simulink model "sm_boom_lift_crawler_test_jib_hydr_1D"  (R2026a)
settings: Solver=ode23t  StopTime=tVec.StopTime  MaxStep=2  AbsTol=1e-4
PostLoadFcn:
  | sm_boom_lift_crawler_settest('jib test')
StartFcn:
  | tic;
StopFcn:
  | Elapsed_Sim_Time = toc;
  | %disp(['Elapsed Sim Time = ' num2str(Elapsed_Sim_Time)]);
undefined symbols (not defined in the file): oVec, tVec
libraries: fl_lib x9, nesl_utility x6, sdl_lib x1, sm_boom_lift_crawler_lib_actuators x1, sm_boom_lift_crawler_lib x1
Description:
  | Copyright 2025-2026 The MathWorks, Inc.
settings Model: Creator=smiller  LastModifiedBy=smiller
settings SolverCC: MaxConsecutiveMinStep=5
settings DataIOCC: SignalLoggingName=logsout_sm_boom_lift_crawler
settings SimscapeCC: SimscapeNominalValues="[{\"value\":\"1\",\"unit\":\"A\"},{\"value\":\"nomval_psi\",\"unit\":\"psi\"},{\"value\":\"1\",\"unit\":\"cm^2\"},{\"value\":\"nomval_cmv3_s\",\"unit\":\"cm^3/s\"},{\"value\":\"1\",\"unit\":\"kJ/kg\"},{\"value\":\"1\",\"unit\":\"kW\"},{\"value\":\"1\",\"unit\":\"l\"},{\"value\":\"nomval_N\",\"unit\":\"N\"},{\"value\":\"nomval_Nm\",\"unit\":\"N*m\"},{\"value\":\"1\",\"unit\":\"V\"}]"  SimscapeLogName=simlog_sm_boom_lift_crawler  SimscapeLogLimitData=off  SimscapeLogDataHistory=5000.0  SimscapeUseOperatingPoints=on  SimscapeOperatingPoint=op_jib_hydr_1D

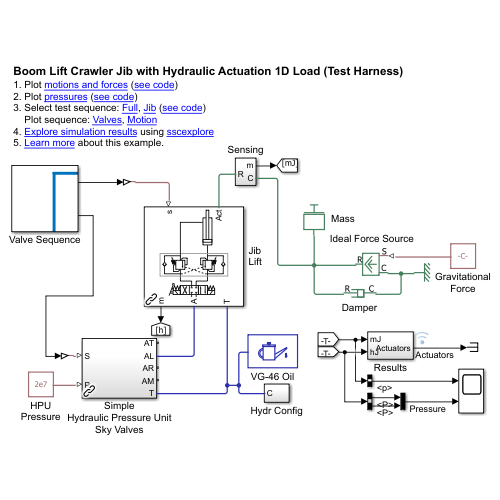
[thumbnail: Simulink's stored preview of the top-level diagram]
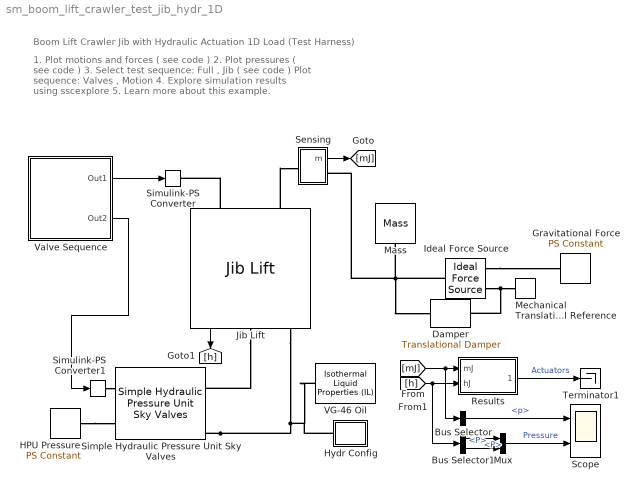
== system sm_boom_lift_crawler_test_jib_hydr_1D ==
  note: Boom Lift Crawler Jib with Hydraulic Actuation 1D Load (Test Harness)
  note: 1. Plot motions and forces ( see code )
      | 2. Plot pressures ( see code )
      | 3. Select test sequence: Full , Jib ( see code )
      | Plot sequence: Valves , Motion
      | 4. Explore simulation results using sscexplore
      | 5. Learn more about this example.
  Bus Selector : BusSelector  OutputSignals=p
  Bus Selector1 : BusSelector  OutputSignals=A.P,B.P
  Damper : sdl_lib/Couplings & Drives/Springs & Dampers/Translational Damper  D=100 N/(m/s)  thermal_port=simscape.enum.thermaleffects.omit  thermal_mass=50 kJ/K  temperature_specify=off  temperature_priority=High  temperature=300 K  temperature_nominal_specify=off  temperature_nominal_value=1  temperature_nominal_unit=K
  Gravitational Force : fl_lib/Physical Signals/Sources/PS Constant  constant=9.8*163
  HPU Pressure : fl_lib/Physical Signals/Sources/PS Constant  constant=2e7 Pa
  Hydr Config : Subsystem
  Ideal Force Source : fl_lib/Mechanical/Mechanical Sources/Ideal Force Source
  Jib Lift : sm_boom_lift_crawler_lib_actuators/Actuators/Sky Manifold/Sky Valves II/Jib Lift  SystemSampleTime=-1  VariantActivationTime=update diagram  EmptyChoice=off  PassThrough=off  PassThroughVariantControl=(default)  EmptyChoiceVariantControl=(default)  AllowFlexibleInterface=on  Latency=0  AutoFrameSizeCalculation=off
  Mass : fl_lib/Mechanical/Translational Elements/Mass  mass=163 kg  num_ports=foundation.enum.numPorts2.one  v_specify=off  v_priority=High  v=0 m/s  v_nominal_specify=off  v_nominal_value=1  v_nominal_unit=m/s  f_specify=off  f_priority=None  f=0 N  f_nominal_specify=off  f_nominal_value=1  f_nominal_unit=N
  Mechanical Translational Reference : fl_lib/Mechanical/Translational Elements/Mechanical Translational Reference
  Mux : Mux  Inputs=2
  Results : Subsystem
  Scope : Scope  NumInputPorts=2
      settings: ActiveDisplayYMinimum=-0.05926  ActiveDisplayYMaximum=0.46698
  Sensing : Subsystem
  Simple Hydraulic Pressure Unit Sky Valves : sm_boom_lift_crawler_lib/Simple Hydraulic Pressure Unit Sky Valves  SystemSampleTime=-1  VariantActivationTime=update diagram  EmptyChoice=off  PassThrough=off  PassThroughVariantControl=(default)  EmptyChoiceVariantControl=(default)  AllowFlexibleInterface=on  Latency=0  AutoFrameSizeCalculation=off
  Simulink-PS Converter : nesl_utility/Simulink-PS Converter  PhysicalDomain=network_engine_domain  SubClassName=ps_input  LeftPortType=input  RightPortType=output  PseudoPeriodic=off  Frequencies=[]  NoiseDistribution=none  NoiseParameters=[]  Unit=1  AffineConversion=off  FilteringAndDerivatives=provide  SimscapeFilterOrder=1  InputFilterTimeConstant=0.001  UdotUserProvided=0
  Simulink-PS Converter1 : nesl_utility/Simulink-PS Converter  PhysicalDomain=network_engine_domain  SubClassName=ps_input  LeftPortType=input  RightPortType=output  PseudoPeriodic=off  Frequencies=[]  NoiseDistribution=none  NoiseParameters=[]  Unit=1  AffineConversion=off  FilteringAndDerivatives=provide  SimscapeFilterOrder=1  InputFilterTimeConstant=0.001  UdotUserProvided=0
  Terminator1 : Terminator
  VG-46 Oil : fl_lib/Isothermal Liquid/Utilities/Isothermal Liquid Properties (IL)  rho_L_atm=867.346 kg/m^3  bulk_modulus_model=foundation.enum.bulk_modulus_model.const  beta_gain=6  beta_L_atm=1.48150e+09 Pa  nu_atm=(45.7333)*(1) cSt  p_atm=0.101325 MPa  p_min=1 Pa  properties_range_check=simscape.enum.assert.action.error  air_fraction=ratio_dissolved_air  polytropic_index=1.0  rho_g_atm=1.225 kg/m^3  air_dissolution_model=simscape.enum.onoff.off  p_crit=3 MPa
  Valve Sequence : Subsystem
      mask Display: image('sm_boom_lift_crawler_valve_seq_outputonly.svg');
  wires:
  [h] -> Bus Selector1/1, Results/2(hJ)
  Valve Sequence/2(Out2) -> Simulink-PS Converter1/1
  Valve Sequence/1(Out1) -> Simulink-PS Converter/1
  Mux/1 -> Scope/2  "Pressure"
  Bus Selector1/2 -> Mux/2  "<P>"
  Sensing/1(m) -> [mJ]
  Bus Selector1/1 -> Mux/1  "<P>"
  [mJ] -> Bus Selector/1, Results/1(mJ)
  Results/1(Actuators) -> Terminator1/1  "Actuators"
  Jib Lift/1 -> [h]
  Bus Selector/1 -> Scope/1  "<p>"
  connections:
  Ideal Force Source/LConn1 -- Mass/LConn1 -- Sensing/RConn1 -- Damper/LConn1
  Mechanical Translational Reference/LConn1 -- Ideal Force Source/RConn2 -- Damper/RConn1
  Simple Hydraulic Pressure Unit Sky Valves/RConn5 -- Jib Lift/RConn2 -- VG-46 Oil/RConn1 -- Hydr Config/RConn1
  Ideal Force Source/RConn1 -- Gravitational Force/RConn1
  HPU Pressure/RConn1 -- Simple Hydraulic Pressure Unit Sky Valves/LConn2
  Simulink-PS Converter1/RConn1 -- Simple Hydraulic Pressure Unit Sky Valves/LConn1
  Jib Lift/RConn1 -- Simple Hydraulic Pressure Unit Sky Valves/RConn2
  Jib Lift/LConn2 -- Sensing/LConn1
  Jib Lift/LConn1 -- Simulink-PS Converter/RConn1

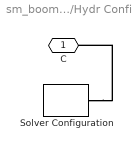
== system sm_boom_lift_crawler_test_jib_hydr_1D/Hydr Config ==
  Solver Configuration : nesl_utility/Solver Configuration  PhysicalDomain=network_engine_domain  SubClassName=solver  LeftPortType=input  RightPortType=generic  Tones=[]  Harmonics=[]  SimulateNoise=off  Profile=off  UseLocalSampling=off  EnableSwitchedLinearOptims=on  FrequencyDomain=off  UseCCode=off  RelTol=0.001  AbsTol=1e-06  MinStep=1e-09  ToWorkspace=off  RevertToSquareIcSolve=off  NumHomotopyIterations=100  PhasorMode=off  PhasorModeNumHarmonics=1  ConsistencySolver=NEWTON_FTOL  CanonicalOrdering=UNORDERED  OptimizeIntermediates=UNOPTIMIZED  IndexReductionMethod=DerivativeReplacement  DoDC=off  ResidualTolerance=1e-9  ConsistencyTolSource=GLOBAL  ConsistencyAbsTol=0.001  ConsistencyRelTol=0.001  ConsistencyTolFactor=0.001  UseLocalSolver=off  LocalSolverChoice=NE_BACKWARD_EULER_ADVANCER  ResolveIndetEquations=on  FunctionEvalNumThread=1  LocalSolverSampleTime=2e-3  DoFixedCost=off  MaxNonlinIter=5  MaxModeIter=2  ComputeImpulses=off  ImpulseIterations=2  LinearAlgebra=Sparse  LinearAlgebraNumThread=0  EquationFormulation=NE_TIME_EF  DelaysMemoryBudget=1024  AutomaticFiltering=on  FilteringTimeConstant=1e-3  PartitionStorageMethod=EXHAUSTIVE  PartitionMemoryBudget=1024  PartitionMethod=FAST  MultibodyUseLocalSolver=off  MultibodyLocalSolverChoice=ODE1  MultibodyLocalSolverSampleTime=0.001
  C : PMIOPort  Side=Right
  connections:
  Solver Configuration/RConn1 -- C/RConn1

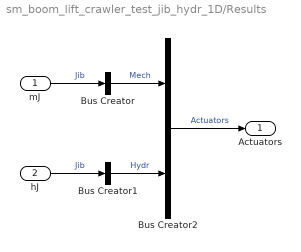
== system sm_boom_lift_crawler_test_jib_hydr_1D/Results ==
  mJ : Inport
  hJ : Inport  Port=2
  Bus Creator : BusCreator  Inputs=1
  Bus Creator1 : BusCreator  Inputs=1
  Bus Creator2 : BusCreator  Inputs=2
  Actuators : Outport
  wires:
  Bus Creator/1 -> Bus Creator2/1  "Mech"
  Bus Creator1/1 -> Bus Creator2/2  "Hydr"
  hJ/1 -> Bus Creator1/1  "Jib"
  mJ/1 -> Bus Creator/1  "Jib"
  Bus Creator2/1 -> Actuators/1  "Actuators"

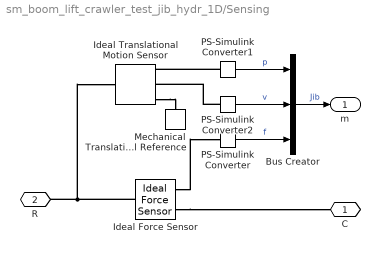
== system sm_boom_lift_crawler_test_jib_hydr_1D/Sensing ==
  Bus Creator : BusCreator  Inputs=3
  Ideal Force Sensor : fl_lib/Mechanical/Mechanical Sensors/Ideal Force Sensor
  Ideal Translational Motion Sensor : fl_lib/Mechanical/Mechanical Sensors/Ideal Translational Motion Sensor  reference=foundation.enum.MeasurementReference.difference  acceleration_port=false  velocity_port=true  position_port=true  offset=0 m
  Mechanical Translational Reference : fl_lib/Mechanical/Translational Elements/Mechanical Translational Reference
  PS-Simulink Converter : nesl_utility/PS-Simulink Converter  PhysicalDomain=network_engine_domain  SubClassName=ps_output  LeftPortType=input  RightPortType=output  PseudoPeriodic=off  Frequencies=[]  VectorFormat=1-D array  Unit=inherit  AffineConversion=off
  PS-Simulink Converter1 : nesl_utility/PS-Simulink Converter  PhysicalDomain=network_engine_domain  SubClassName=ps_output  LeftPortType=input  RightPortType=output  PseudoPeriodic=off  Frequencies=[]  VectorFormat=1-D array  Unit=inherit  AffineConversion=off
  PS-Simulink Converter2 : nesl_utility/PS-Simulink Converter  PhysicalDomain=network_engine_domain  SubClassName=ps_output  LeftPortType=input  RightPortType=output  PseudoPeriodic=off  Frequencies=[]  VectorFormat=1-D array  Unit=inherit  AffineConversion=off
  C : PMIOPort  Side=Right
  R : PMIOPort  Port=2  Side=Left
  m : Outport
  wires:
  PS-Simulink Converter2/1 -> Bus Creator/2  "v"
  PS-Simulink Converter/1 -> Bus Creator/3  "f"
  PS-Simulink Converter1/1 -> Bus Creator/1  "p"
  Bus Creator/1 -> m/1  "Jib"
  connections:
  Ideal Force Sensor/RConn2 -- PS-Simulink Converter/LConn1
  Ideal Force Sensor/LConn1 -- R/RConn1 -- Ideal Translational Motion Sensor/LConn1
  Ideal Force Sensor/RConn1 -- C/RConn1
  Ideal Translational Motion Sensor/RConn1 -- Mechanical Translational Reference/LConn1
  PS-Simulink Converter1/LConn1 -- Ideal Translational Motion Sensor/RConn3
  PS-Simulink Converter2/LConn1 -- Ideal Translational Motion Sensor/RConn2

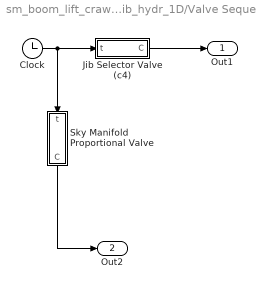
== system sm_boom_lift_crawler_test_jib_hydr_1D/Valve Sequence ==
  Clock : Clock
  Jib Selector Valve (c4) : Subsystem
  Sky Manifold Proportional Valve : Subsystem
  Out1 : Outport
  Out2 : Outport  Port=2
  wires:
  Sky Manifold Proportional Valve/1(C) -> Out2/1
  Clock/1 -> Jib Selector Valve (c4)/1(t), Sky Manifold Proportional Valve/1(t)
  Jib Selector Valve (c4)/1(C) -> Out1/1

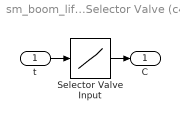
== system sm_boom_lift_crawler_test_jib_hydr_1D/Valve Sequence/Jib Selector Valve (c4) ==
  t : Inport
  Selector Valve Input : Lookup_n-D  NumberOfTableDimensions=1  BreakpointsForDimension1=tVec.sky.c4.all  Table=oVec.sky.c4.all  InterpMethod=Flat  ExtrapMethod=Clip  UseLastTableValue=on  InternalRulePriority=Speed  RndMeth=Simplest
  C : Outport
  wires:
  Selector Valve Input/1 -> C/1
  t/1 -> Selector Valve Input/1

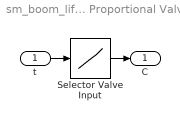
== system sm_boom_lift_crawler_test_jib_hydr_1D/Valve Sequence/Sky Manifold Proportional Valve ==
  t : Inport
  Selector Valve Input : Lookup_n-D  NumberOfTableDimensions=1  BreakpointsForDimension1=tVec.sky.proportional  Table=oVec.sky.proportional  InterpMethod=Flat  ExtrapMethod=Clip  UseLastTableValue=on  InternalRulePriority=Speed  RndMeth=Simplest
  C : Outport
  wires:
  t/1 -> Selector Valve Input/1
  Selector Valve Input/1 -> C/1
